simulink model "uas_sim"  (R2020b)
settings: Solver=VariableStepAuto  StartTime=0.0  StopTime=10.0  RelTol=1e-3
undefined symbols (not defined in the file or in its folder): b, c, Earth, InitCond, prop_angle, voltage, WGS84
libraries: aerolibasang x3, aerolibactuator x1, aerolibadyn x1, sharedutil x1, aerolibbdyn x1, sharedtransform x1, shared6dof x1, aerolibconvert2 x1, aerolibtransform2 x1, aerolibgravity2 x1
settings Model: Creator=brian  LastModifiedBy=brian

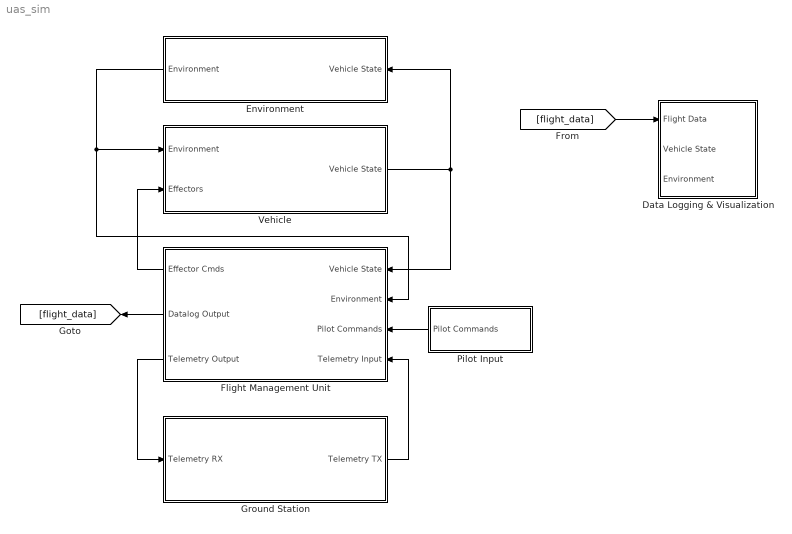
== system uas_sim ==
  Data Logging & Visualization : Subsystem
  Environment : Subsystem
  Flight Management Unit : Subsystem
  Ground Station : Subsystem
  Pilot Input : Subsystem
  Vehicle : Subsystem
  wires:
  Vehicle/1(Vehicle State) -> Flight Management Unit/1(Vehicle State), Environment/1(Vehicle State)
  Pilot Input/1(Pilot Commands) -> Flight Management Unit/3(Pilot Commands)
  Ground Station/1(Telemetry TX) -> Flight Management Unit/4(Telemetry Input)
  Flight Management Unit/3(Telemetry Output) -> Ground Station/1(Telemetry RX)
  Flight Management Unit/1(Effector Cmds) -> Vehicle/2(Effectors)
  [flight_data] -> Data Logging & Visualization/1(Flight Data)
  Flight Management Unit/2(Datalog Output) -> [flight_data]
  Environment/1(Environment) -> Vehicle/1(Environment), Flight Management Unit/2(Environment)

== system uas_sim/Data Logging & Visualization ==
  Flight Data : Inport
  Vehicle State : Inport  Port=2
  Environment : Inport  Port=3

== system uas_sim/Environment ==
  Vehicle State : Inport
  Bus Creator : BusCreator  Inputs=6
  Bus Selector : BusSelector  OutputSignals=Latitude [rad],Longitude [rad],Altitude WGS84 [m]
  Model : ModelReference  ModelNameDialog=env_mdl_aero_blockset.slx  SimulationMode=Normal  ModelReferenceVersion=1.5
  Environment : Outport
  wires:
  Vehicle State/1 -> Bus Selector/1
  Bus Selector/1 -> Model/1  "<Latitude [rad]>"
  Bus Selector/2 -> Model/2  "<Longitude [rad]>"
  Bus Selector/3 -> Model/3  "<Altitude WGS84 [m]>"
  Bus Creator/1 -> Environment/1
  Model/3 -> Bus Creator/3  "Pressure [Pa]"
  Model/2 -> Bus Creator/2  "Speed of Sound [m/s]"
  Model/1 -> Bus Creator/1  "Temperature [K]"
  Model/4 -> Bus Creator/4  "Density [kg/m^3]"
  Model/5 -> Bus Creator/5  "Gravity [m/s/s]"
  Model/6 -> Bus Creator/6  "Magnetic Field [uT]"

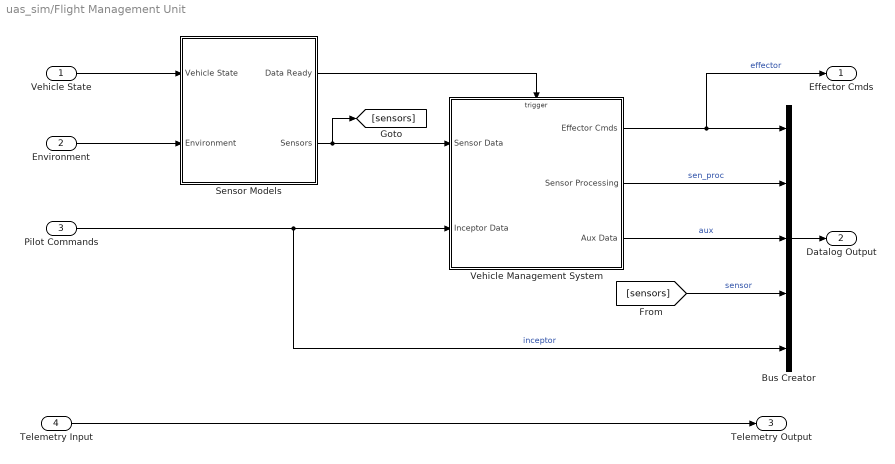
== system uas_sim/Flight Management Unit ==
  Vehicle State : Inport
  Environment : Inport  Port=2
  Pilot Commands : Inport  Port=3  OutDataTypeStr=Bus: InceptorData
  Telemetry Input : Inport  Port=4
  Bus Creator : BusCreator  Inputs=5
  Sensor Models : Subsystem
      settings: PortSchema="{\"entries\":[{\"content\":{\"sides\":[{\"content\":{\"connectorIds\":[]},\"type\":\"ConnectorPlacement.EquallySpacedRectSide\",\"uuid\":\"b20f7590-d69b-48b8-beb1-2fb7d3ab0357\"},{\"content\":{\"connectorIds\":[],\"side\":\"RIGHT\"},\"type\":\"ConnectorPlacement.EquallySpacedRectSide\",\"uuid\":\"07801f8a-7756-483e-a050-3c2fccc33404\"},{\"content\":{\"connectorIds\":[\"In1\",\"In2\"],\"side\":\"TOP\"},\"type\":\"ConnectorPlacement.EquallySpacedRectSide\",\"uuid\":\"ce3c3c94-ed36-4103-b079-69dcaeaf21e9\"},{\"content\":{\"connectorIds\":[\"Out1\",\"Out2\"],\"side\":\"BOTTOM\"},\"type\":\"ConnectorPlacement.EquallySpacedRectSide\",\"uuid\":\"ba78b819-a471-4bc3-b479-e6a973cfe14f\"},{\"content\":{\"connectorIds\":[],\"side\":\"HIDDEN\"},\"type\":\"ConnectorPlacement.EquallySpacedRectSide\",\"uuid\":\"3cf915a5-25a1-4380-9090-9561533312da\"}]},\"type\":\"ConnectorPlacement.EquallySpacedConnector\",\"uuid\":\"7ef4ddaa-ccd2-4778-89ce-8b4685524e82\"}],\"packageUris\":[\"http://schema.mathworks.com/mf0/Connector/R2020b\"],\"version\":\"1.0\"}"
  Vehicle Management System : Subsystem  TreatAsAtomicUnit=on
  Effector Cmds : Outport  OutDataTypeStr=Bus: EffectorCmds
  Datalog Output : Outport  Port=2
  Telemetry Output : Outport  Port=3
  wires:
  Telemetry Input/1 -> Telemetry Output/1
  Pilot Commands/1 -> Bus Creator/5, Vehicle Management System/2(Inceptor Data)  "inceptor"
  Sensor Models/2(Data Ready) -> Vehicle Management System/Trigger
  Bus Creator/1 -> Datalog Output/1
  Vehicle Management System/3(Aux Data) -> Bus Creator/3  "aux"
  Vehicle Management System/1(Effector Cmds) -> Effector Cmds/1, Bus Creator/1  "effector"
  Vehicle Management System/2(Sensor Processing) -> Bus Creator/2  "sen_proc"
  Environment/1 -> Sensor Models/1(Environment)
  Vehicle State/1 -> Sensor Models/2(Vehicle State)
  Sensor Models/1(Sensors) -> [sensors], Vehicle Management System/1(Sensor Data)
  [sensors] -> Bus Creator/4  "sensor"

== system uas_sim/Ground Station ==
  Telemetry RX : Inport
  Telemetry TX : Outport
  wires:
  Telemetry RX/1 -> Telemetry TX/1

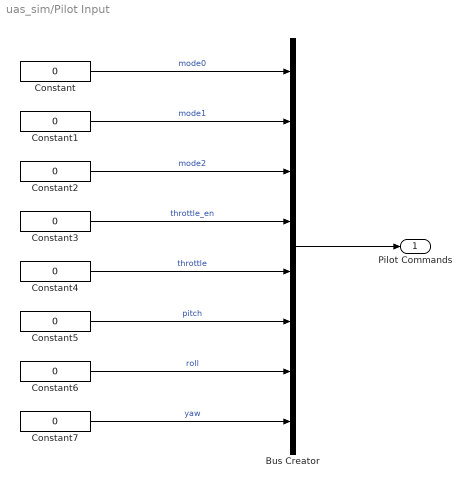
== system uas_sim/Pilot Input ==
  Bus Creator : BusCreator  Inputs=8
  Constant{,1..7} (8 alike) : Constant  Value=0
  Pilot Commands : Outport  OutDataTypeStr=Bus: InceptorData
  wires:
  Bus Creator/1 -> Pilot Commands/1
  Constant/1 -> Bus Creator/1  "mode0"
  Constant1/1 -> Bus Creator/2  "mode1"
  Constant2/1 -> Bus Creator/3  "mode2"
  Constant3/1 -> Bus Creator/4  "throttle_en"
  Constant4/1 -> Bus Creator/5  "throttle"
  Constant5/1 -> Bus Creator/6  "pitch"
  Constant6/1 -> Bus Creator/7  "roll"
  Constant7/1 -> Bus Creator/8  "yaw"

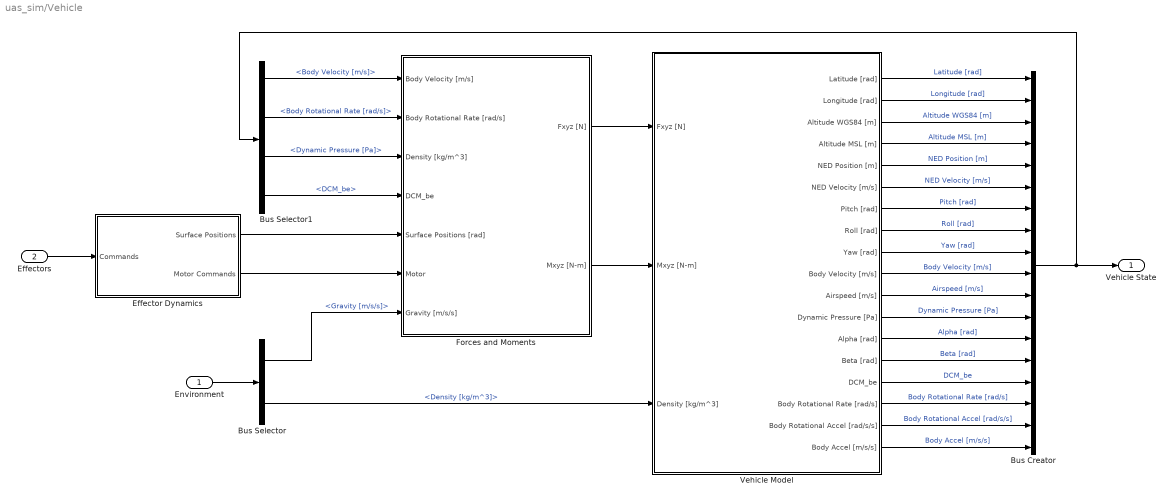
== system uas_sim/Vehicle ==
  Environment : Inport
  Effectors : Inport  Port=2
  Bus Creator : BusCreator  Inputs=18
  Bus Selector : BusSelector  OutputSignals=Gravity [m/s/s],Density [kg/m^3]
  Bus Selector1 : BusSelector  OutputSignals=Body Velocity [m/s],Body Rotational Rate [rad/s],Dynamic Pressure [Pa],DCM_be
  Effector Dynamics : Subsystem
      settings: PortSchema="{\"entries\":[{\"content\":{\"sides\":[{\"content\":{\"connectorIds\":[]},\"type\":\"ConnectorPlacement.EquallySpacedRectSide\",\"uuid\":\"b20f7590-d69b-48b8-beb1-2fb7d3ab0357\"},{\"content\":{\"connectorIds\":[],\"side\":\"RIGHT\"},\"type\":\"ConnectorPlacement.EquallySpacedRectSide\",\"uuid\":\"07801f8a-7756-483e-a050-3c2fccc33404\"},{\"content\":{\"connectorIds\":[\"Out1\",\"Out2\"],\"side\":\"TOP\"},\"type\":\"ConnectorPlacement.EquallySpacedRectSide\",\"uuid\":\"ce3c3c94-ed36-4103-b079-69dcaeaf21e9\"},{\"content\":{\"connectorIds\":[\"In1\"],\"side\":\"BOTTOM\"},\"type\":\"ConnectorPlacement.EquallySpacedRectSide\",\"uuid\":\"ba78b819-a471-4bc3-b479-e6a973cfe14f\"},{\"content\":{\"connectorIds\":[],\"side\":\"HIDDEN\"},\"type\":\"ConnectorPlacement.EquallySpacedRectSide\",\"uuid\":\"3cf915a5-25a1-4380-9090-9561533312da\"}]},\"type\":\"ConnectorPlacement.EquallySpacedConnector\",\"uuid\":\"7ef4ddaa-ccd2-4778-89ce-8b4685524e82\"}],\"packageUris\":[\"http://schema.mathworks.com/mf0/Connector/R2020b\"],\"version\":\"1.0\"}"
  Forces and Moments : Subsystem
  Vehicle Model : Subsystem
  Vehicle State : Outport
  wires:
  Vehicle Model/1(Latitude [rad]) -> Bus Creator/1  "Latitude [rad]"
  Vehicle Model/2(Longitude [rad]) -> Bus Creator/2  "Longitude [rad]"
  Vehicle Model/3(Altitude WGS84 [m]) -> Bus Creator/3  "Altitude WGS84 [m]"
  Vehicle Model/4(Altitude MSL [m]) -> Bus Creator/4  "Altitude MSL [m]"
  Vehicle Model/5(NED Position [m]) -> Bus Creator/5  "NED Position [m]"
  Vehicle Model/6(NED Velocity [m/s]) -> Bus Creator/6  "NED Velocity [m/s]"
  Vehicle Model/7(Pitch [rad]) -> Bus Creator/7  "Pitch [rad]"
  Vehicle Model/8(Roll [rad]) -> Bus Creator/8  "Roll [rad]"
  Vehicle Model/9(Yaw [rad]) -> Bus Creator/9  "Yaw [rad]"
  Vehicle Model/12(Dynamic Pressure [Pa]) -> Bus Creator/12  "Dynamic Pressure [Pa]"
  Vehicle Model/13(Alpha [rad]) -> Bus Creator/13  "Alpha [rad]"
  Vehicle Model/14(Beta [rad]) -> Bus Creator/14  "Beta [rad]"
  Vehicle Model/15(DCM_be) -> Bus Creator/15  "DCM_be"
  Vehicle Model/16(Body Rotational Rate [rad/s]) -> Bus Creator/16  "Body Rotational Rate [rad/s]"
  Vehicle Model/17(Body Rotational Accel [rad/s/s]) -> Bus Creator/17  "Body Rotational Accel [rad/s/s]"
  Vehicle Model/18(Body Accel [m/s/s]) -> Bus Creator/18  "Body Accel [m/s/s]"
  Effectors/1 -> Effector Dynamics/1(Commands)
  Effector Dynamics/1(Surface Positions) -> Forces and Moments/5(Surface Positions [rad])
  Effector Dynamics/2(Motor Commands) -> Forces and Moments/6(Motor)
  Environment/1 -> Bus Selector/1
  Bus Selector/1 -> Forces and Moments/7(Gravity [m/s/s])  "<Gravity [m/s/s]>"
  Bus Selector/2 -> Vehicle Model/3(Density [kg/m^3])  "<Density [kg/m^3]>"
  Bus Creator/1 -> Bus Selector1/1, Vehicle State/1
  Vehicle Model/11(Airspeed [m/s]) -> Bus Creator/11  "Airspeed [m/s]"
  Bus Selector1/4 -> Forces and Moments/4(DCM_be)  "<DCM_be>"
  Vehicle Model/10(Body Velocity [m/s]) -> Bus Creator/10  "Body Velocity [m/s]"
  Bus Selector1/1 -> Forces and Moments/1(Body Velocity [m/s])  "<Body Velocity [m/s]>"
  Bus Selector1/2 -> Forces and Moments/2(Body Rotational Rate [rad/s])  "<Body Rotational Rate [rad/s]>"
  Bus Selector1/3 -> Forces and Moments/3(Density [kg/m^3])  "<Dynamic Pressure [Pa]>"
  Forces and Moments/1(Fxyz [N]) -> Vehicle Model/1(Fxyz [N])
  Forces and Moments/2(Mxyz [N-m]) -> Vehicle Model/2(Mxyz [N-m])

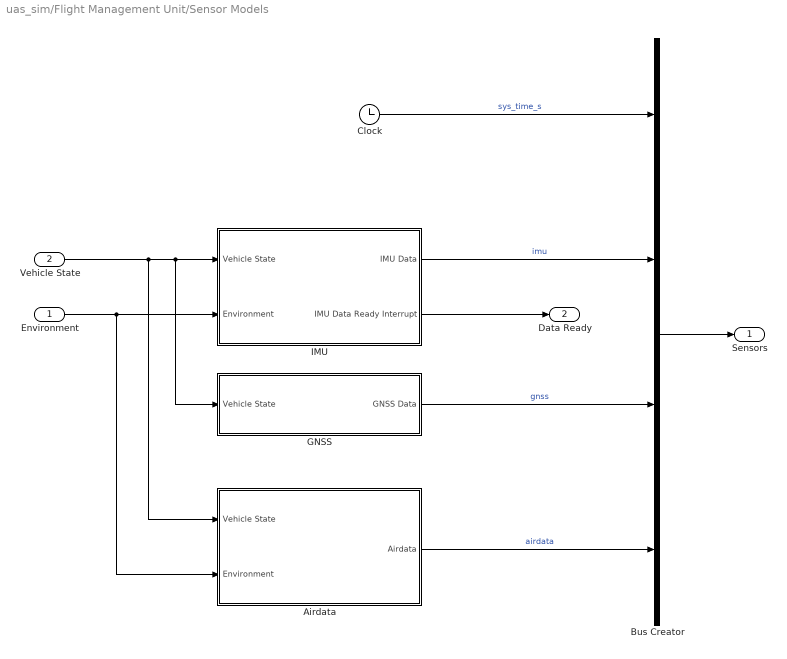
== system uas_sim/Flight Management Unit/Sensor Models ==
  Environment : Inport
  Vehicle State : Inport  Port=2
  Airdata : Subsystem
  Bus Creator : BusCreator  Inputs=4  OutDataTypeStr=Bus: SensorData  NonVirtualBus=on
      settings: InheritFromInputs=off
  Clock : Clock
      settings: Decimation=1e6
  GNSS : Subsystem
  IMU : Subsystem
  Sensors : Outport
  Data Ready : Outport  Port=2
  wires:
  Bus Creator/1 -> Sensors/1
  Clock/1 -> Bus Creator/1  "sys_time_s"
  IMU/1(IMU Data) -> Bus Creator/2  "imu"
  IMU/2(IMU Data Ready Interrupt) -> Data Ready/1
  Vehicle State/1 -> Airdata/1(Vehicle State), GNSS/1(Vehicle State), IMU/1(Vehicle State)
  Environment/1 -> Airdata/2(Environment), IMU/2(Environment)
  GNSS/1(GNSS Data) -> Bus Creator/3  "gnss"
  Airdata/1(Airdata) -> Bus Creator/4  "airdata"

== system uas_sim/Flight Management Unit/Vehicle Management System ==
  Sensor Data : Inport  OutDataTypeStr=Bus: SensorData
  Inceptor Data : Inport  Port=2  OutDataTypeStr=Bus: SenProcData
  Trigger : TriggerPort  VariantControl=Variant
  Model : ModelReference  ModelNameDialog=baseline.slx  SimulationMode=Normal  ModelReferenceVersion=1.11
  Effector Cmds : Outport  OutDataTypeStr=Bus: EffectorCmds
  Sensor Processing : Outport  Port=2  OutDataTypeStr=Bus: SenProcData
  Aux Data : Outport  Port=3  OutDataTypeStr=Bus: AuxData
  wires:
  Model/2 -> Sensor Processing/1
  Model/3 -> Aux Data/1
  Model/1 -> Effector Cmds/1
  Sensor Data/1 -> Model/1
  Inceptor Data/1 -> Model/2

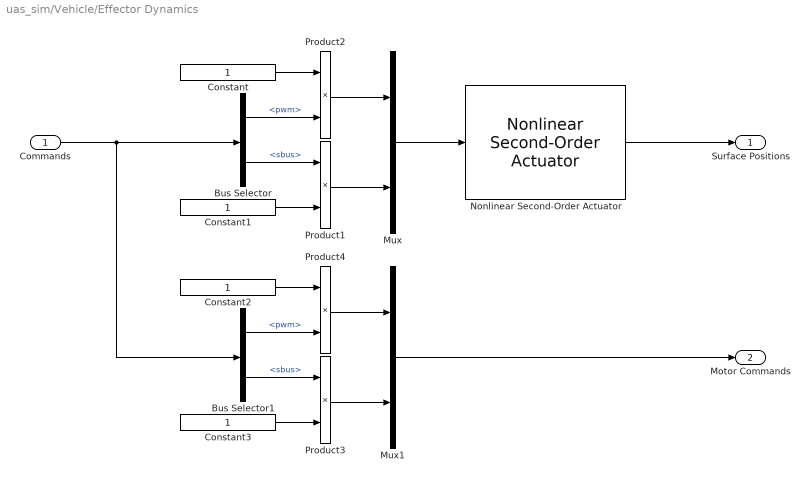
== system uas_sim/Vehicle/Effector Dynamics ==
  Commands : Inport
  Bus Selector : BusSelector  OutputSignals=pwm,sbus
  Bus Selector1 : BusSelector  OutputSignals=pwm,sbus
  Constant{,1..3} (4 alike) : Constant
  Mux : Mux  Inputs=2
  Mux1 : Mux  Inputs=2
  Nonlinear Second-Order Actuator : aerolibactuator/Nonlinear Second-Order Actuator  wn_fin=1  z_fin=0.3  fin_max=20*pi/180  fin_min=-20*pi/180  fin_maxrate=500*pi/180  fin_act_0=0  fin_act_vel=0
      settings: SourceProductBaseCode=AE
  Product{1..4} (4 alike) : Product
  Surface Positions : Outport
  Motor Commands : Outport  Port=2
  wires:
  Commands/1 -> Bus Selector1/1, Bus Selector/1
  Bus Selector/1 -> Product2/2  "<pwm>"
  Bus Selector/2 -> Product1/1  "<sbus>"
  Mux/1 -> Nonlinear Second-Order Actuator/1
  Nonlinear Second-Order Actuator/1 -> Surface Positions/1
  Product2/1 -> Mux/1
  Product1/1 -> Mux/2
  Constant/1 -> Product2/1
  Constant1/1 -> Product1/2
  Constant3/1 -> Product3/2
  Constant2/1 -> Product4/1
  Product3/1 -> Mux1/2
  Product4/1 -> Mux1/1
  Mux1/1 -> Motor Commands/1
  Bus Selector1/2 -> Product3/1  "<sbus>"
  Bus Selector1/1 -> Product4/2  "<pwm>"

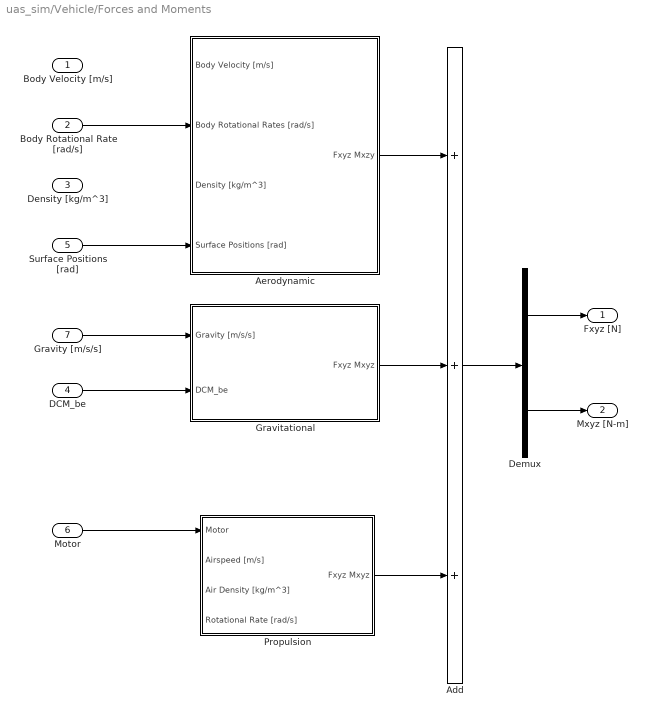
== system uas_sim/Vehicle/Forces and Moments ==
  Body Velocity [m/s] : Inport
  Body Rotational Rate [rad/s] : Inport  Port=2
  Density [kg/m^3] : Inport  Port=3
  DCM_be : Inport  Port=4
  Surface Positions [rad] : Inport  Port=5
  Motor : Inport  Port=6
  Gravity [m/s/s] : Inport  Port=7
  Add : Sum  Inputs=+++
  Aerodynamic : Subsystem
  Demux : Demux  Outputs=2
  Gravitational : Subsystem
  Propulsion : Subsystem
  Fxyz [N] : Outport
  Mxyz [N-m] : Outport  Port=2
  wires:
  Surface Positions [rad]/1 -> Aerodynamic/4(Surface Positions [rad])
  Body Rotational Rate [rad/s]/1 -> Aerodynamic/2(Body Rotational Rates [rad/s])
  Gravitational/1(Fxyz Mxyz) -> Add/2
  Aerodynamic/1(Fxyz Mxzy) -> Add/1
  Propulsion/1(Fxyz Mxyz) -> Add/3
  Gravity [m/s/s]/1 -> Gravitational/1(Gravity [m/s/s])
  DCM_be/1 -> Gravitational/2(DCM_be)
  Motor/1 -> Propulsion/1(Motor)
  Add/1 -> Demux/1
  Demux/2 -> Mxyz [N-m]/1
  Demux/1 -> Fxyz [N]/1

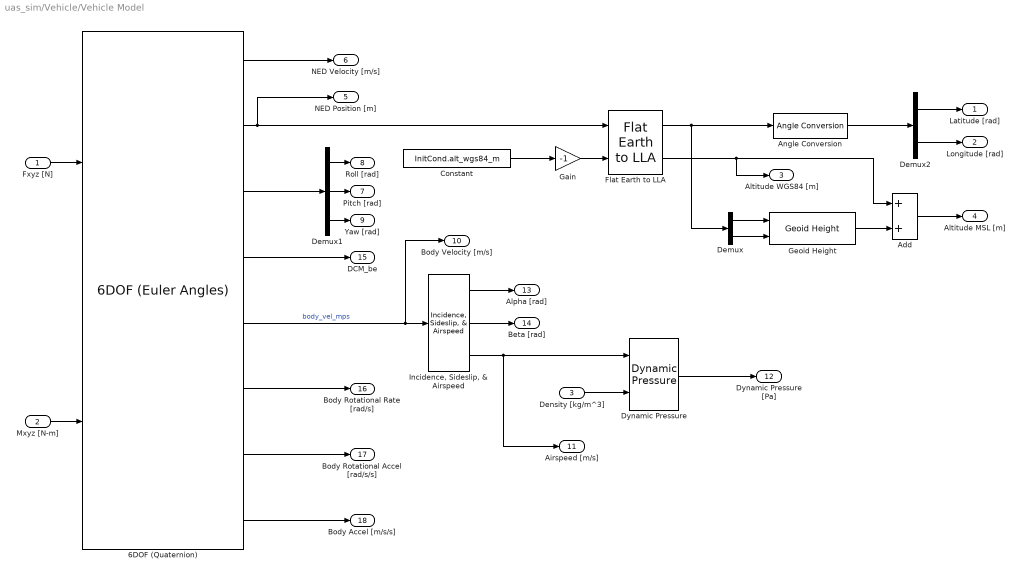
== system uas_sim/Vehicle/Vehicle Model ==
  Fxyz [N] : Inport
  Mxyz [N-m] : Inport  Port=2
  Density [kg/m^3] : Inport  Port=3
  6DOF (Quaternion) : shared6dof/6DOF (Euler Angles)  units=Metric (MKS)  mtype=Fixed  rep=Euler Angles  xme_0=[0 0 0]  Vm_0=[InitCond.vel_u_mps InitCond.vel_v_mps InitCond.vel_w_mps]  eul_0=[InitCond.roll_rad InitCond.pitch_rad InitCond.yaw_rad]  pm_0=[InitCond.p_radps InitCond.q_rads InitCond.r_radps]  mass_0=Aircraft.Mass.mass_kg  mass_e=0.5  mass_f=2.0  inertia=Aircraft.Mass.inertia_kgm2  inertia_e=eye(3)  inertia_f=2*eye(3)  k_quat=1.0  vre_flag=on  abi_flag=off  aMode=0  xme_statename=''  Vm_statename=''  eul_statename=''  quat_statename=''  pm_statename=''  mass_statename=''
      settings: SourceProductBaseCode=AE,PW,MT,UV,VE,VP
  Add : Sum
  Angle Conversion : aerolibconvert2/Angle Conversion  IU=deg  OU=rad
  Constant : Constant  Value=InitCond.alt_wgs84_m
  Demux : Demux  Outputs=2
  Demux1 : Demux  Outputs=3
  Demux2 : Demux  Outputs=2
  Dynamic Pressure : aerolibasang/Dynamic Pressure
  Flat Earth to LLA : aerolibtransform2/Flat Earth to LLA  units=Metric (MKS)  ptype=Earth (WGS84)  F=1/298.257223563  R=6378137  refPosPort=off  LL0=[rad2deg(InitCond.lat_rad) rad2deg(InitCond.lon_rad)]  psi=0
  Gain : Gain  Gain=-1
  Geoid Height : aerolibgravity2/Geoid Height  units=Metric (MKS)  gtype=EGM2008  datafile='geoidegm96grid'  dtype=double  action=Warning
      settings: AttributesFormatString=EGM2008 Geoid Data Unavailable  SourceProductBaseCode=AE
  "Incidence, Sideslip, & Airspeed" : aerolibasang/Incidence, Sideslip, & Airspeed
  Latitude [rad] : Outport
  Longitude [rad] : Outport  Port=2
  Altitude WGS84 [m] : Outport  Port=3
  Altitude MSL [m] : Outport  Port=4
  NED Position [m] : Outport  Port=5
  NED Velocity [m/s] : Outport  Port=6
  Pitch [rad] : Outport  Port=7
  Roll [rad] : Outport  Port=8
  Yaw [rad] : Outport  Port=9
  Body Velocity [m/s] : Outport  Port=10
  Airspeed [m/s] : Outport  Port=11
  Dynamic Pressure [Pa] : Outport  Port=12
  Alpha [rad] : Outport  Port=13
  Beta [rad] : Outport  Port=14
  DCM_be : Outport  Port=15
  Body Rotational Rate [rad/s] : Outport  Port=16
  Body Rotational Accel [rad/s/s] : Outport  Port=17
  Body Accel [m/s/s] : Outport  Port=18
  wires:
  Fxyz [N]/1 -> 6DOF (Quaternion)/1
  Mxyz [N-m]/1 -> 6DOF (Quaternion)/2
  6DOF (Quaternion)/2 -> NED Position [m]/1, Flat Earth to LLA/1
  6DOF (Quaternion)/5 -> Body Velocity [m/s]/1, "Incidence, Sideslip, & Airspeed"/1  "body_vel_mps"
  Flat Earth to LLA/1 -> Demux/1, Angle Conversion/1
  Flat Earth to LLA/2 -> Altitude WGS84 [m]/1, Add/1
  Geoid Height/1 -> Add/2
  Demux/2 -> Geoid Height/2
  Demux/1 -> Geoid Height/1
  "Incidence, Sideslip, & Airspeed"/3 -> Airspeed [m/s]/1, Dynamic Pressure/1
  Density [kg/m^3]/1 -> Dynamic Pressure/2
  Angle Conversion/1 -> Demux2/1
  6DOF (Quaternion)/1 -> NED Velocity [m/s]/1
  6DOF (Quaternion)/4 -> DCM_be/1
  Demux1/1 -> Roll [rad]/1
  6DOF (Quaternion)/3 -> Demux1/1
  Demux1/2 -> Pitch [rad]/1
  Demux1/3 -> Yaw [rad]/1
  Dynamic Pressure/1 -> Dynamic Pressure [Pa]/1
  "Incidence, Sideslip, & Airspeed"/1 -> Alpha [rad]/1
  "Incidence, Sideslip, & Airspeed"/2 -> Beta [rad]/1
  Add/1 -> Altitude MSL [m]/1
  Gain/1 -> Flat Earth to LLA/2
  Constant/1 -> Gain/1
  Demux2/2 -> Longitude [rad]/1
  Demux2/1 -> Latitude [rad]/1
  6DOF (Quaternion)/6 -> Body Rotational Rate [rad/s]/1
  6DOF (Quaternion)/7 -> Body Rotational Accel [rad/s/s]/1
  6DOF (Quaternion)/8 -> Body Accel [m/s/s]/1

== system uas_sim/Flight Management Unit/Sensor Models/Airdata ==
  Vehicle State : Inport
  Environment : Inport  Port=2
  Bus Creator : BusCreator  Inputs=2
  Bus Selector : BusSelector  OutputSignals=Dynamic Pressure [Pa]
  Bus Selector1 : BusSelector  OutputSignals=Pressure [Pa]
  Model : ModelReference  ModelNameDialog=pressure.slx  UsingDefaultArgumentValue=0,0,0,0,0,0  SimulationMode=Normal  ModelReferenceVersion=1.10  scale=Sensors.DiffPres.scale_factor  bias=Sensors.DiffPres.bias_pa  noise=Sensors.DiffPres.noise_pa  p_sath=Sensors.DiffPres.upper_limit_pa  p_satl=Sensors.DiffPres.lower_limit_pa  sample_rate=Sensors.DiffPres.sample_rate_hz  SimulationMode=Normal
  Model1 : ModelReference  ModelNameDialog=pressure.slx  UsingDefaultArgumentValue=0,0,0,0,0,0  SimulationMode=Normal  ModelReferenceVersion=1.10  scale=Sensors.StaticPres.scale_factor  bias=Sensors.StaticPres.bias_pa  noise=Sensors.StaticPres.noise_pa  p_sath=Sensors.StaticPres.upper_limit_pa  p_satl=Sensors.StaticPres.lower_limit_pa  sample_rate=Sensors.StaticPres.sample_rate_hz  SimulationMode=Normal
  Airdata : Outport  OutDataTypeStr=Bus: AirData
  wires:
  Vehicle State/1 -> Bus Selector/1
  Bus Selector/1 -> Model/1  "<Dynamic Pressure [Pa]>"
  Model/1 -> Bus Creator/1  "diff_pres_pa"
  Bus Creator/1 -> Airdata/1
  Model1/1 -> Bus Creator/2  "static_pres_pa"
  Environment/1 -> Bus Selector1/1
  Bus Selector1/1 -> Model1/1  "<Pressure [Pa]>"

== system uas_sim/Flight Management Unit/Sensor Models/GNSS ==
  Vehicle State : Inport
  Bus Creator : BusCreator  Inputs=13  OutDataTypeStr=Bus: GnssData
      settings: InheritFromInputs=off
  Bus Selector : BusSelector  OutputSignals=Latitude [rad],Longitude [rad],Altitude WGS84 [m],NED Velocity [m/s]
  Demux : Demux  Outputs=3
  Model : ModelReference  ModelNameDialog=gnss_receiver.slx  UsingDefaultArgumentValue=0,0,0,0,0  SimulationMode=Normal  ModelReferenceVersion=1.25  fix=Sensors.Gnss.fix  num_sat=Sensors.Gnss.num_satellites  pos_acc_m=Sensors.Gnss.pos_accuracy_m  vel_acc_mps=Sensors.Gnss.vel_accuracy_mps  sample_rate=Sensors.Gnss.sample_rate_hz  SimulationMode=Normal
  GNSS Data : Outport  OutDataTypeStr=Bus: GnssData
  wires:
  Vehicle State/1 -> Bus Selector/1
  Bus Selector/1 -> Model/1  "<Latitude [rad]>"
  Bus Selector/2 -> Model/2  "<Longitude [rad]>"
  Bus Selector/3 -> Model/3  "<Altitude WGS84 [m]>"
  Bus Selector/4 -> Model/4  "<NED Velocity [m/s]>"
  Bus Creator/1 -> GNSS Data/1
  Model/1 -> Bus Creator/1  "fix"
  Model/2 -> Bus Creator/2  "num_sats"
  Model/3 -> Bus Creator/3  "tow_s"
  Model/4 -> Bus Creator/4  "week"
  Model/5 -> Bus Creator/5  "lat_rad"
  Model/6 -> Bus Creator/6  "lon_rad"
  Model/7 -> Bus Creator/7  "alt_wgs84_m"
  Model/11 -> Bus Creator/13  "vel_acc_mps"
  Model/10 -> Bus Creator/12  "vert_acc_m"
  Model/9 -> Bus Creator/11  "horz_acc_m"
  Demux/2 -> Bus Creator/9  "ned_vel_y_mps"
  Demux/1 -> Bus Creator/8  "ned_vel_x_mps"
  Demux/3 -> Bus Creator/10  "ned_vel_z_mps"
  Model/8 -> Demux/1

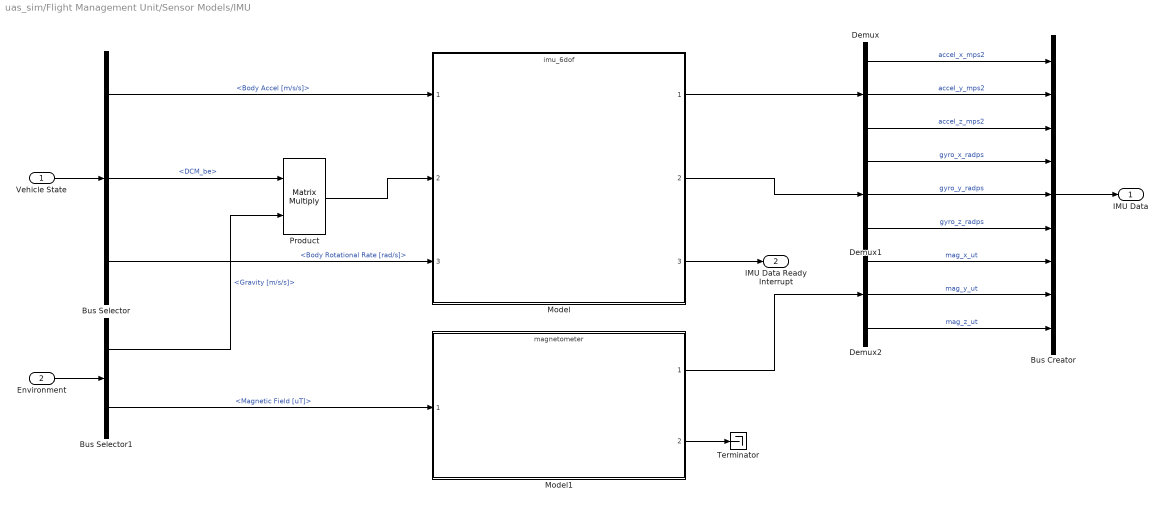
== system uas_sim/Flight Management Unit/Sensor Models/IMU ==
  Vehicle State : Inport
  Environment : Inport  Port=2
  Bus Creator : BusCreator  Inputs=9  OutDataTypeStr=Bus: ImuData
      settings: InheritFromInputs=off
  Bus Selector : BusSelector  OutputSignals=Body Accel [m/s/s],DCM_be,Body Rotational Rate [rad/s]
  Bus Selector1 : BusSelector  OutputSignals=Gravity [m/s/s],Magnetic Field [uT]
  Demux : Demux  Outputs=3
  Demux1 : Demux  Outputs=3
  Demux2 : Demux  Outputs=3
  Model : ModelReference  ModelNameDialog=imu_6dof.slx  UsingDefaultArgumentValue=0,0,0,0,0,0,0,0,0,0,0,0  SimulationMode=Normal  ModelReferenceVersion=1.19  sample_rate=Sensors.Imu.sample_rate_hz  a_sf_cc=Sensors.Imu.Accel.scale_factor  a_bias=Sensors.Imu.Accel.bias_mps2  a_noise=Sensors.Imu.Accel.noise_mps2  a_sath=Sensors.Imu.Accel.upper_limit_mps2  a_satl=Sensors.Imu.Accel.lower_limit_mps2  g_sf_cc=Sensors.Imu.Gyro.scale_factor  g_sen=Sensors.Imu.Gyro.accel_sens_radps  g_bias=Sensors.Imu.Gyro.bias_radps  g_noise=Sensors.Imu.Gyro.noise_radps  g_sath=Sensors.Imu.Gyro.upper_limit_radps  g_satl=Sensors.Imu.Gyro.lower_limit_radps  SimulationMode=Normal
  Model1 : ModelReference  ModelNameDialog=magnetometer.slx  UsingDefaultArgumentValue=0,0,0,0,0,0  SimulationMode=Normal  ModelReferenceVersion=1.24  m_sf_cc=Sensors.Imu.Mag.scale_factor  m_bias=Sensors.Imu.Mag.bias_ut  m_noise=Sensors.Imu.Mag.noise_ut  m_sath=Sensors.Imu.Mag.upper_limit_ut  m_satl=Sensors.Imu.Mag.lower_limit_ut  sample_rate=Sensors.Imu.mag.sample_rate_hz  SimulationMode=Normal
  Product : Product  Multiplication=Matrix(*)
  Terminator : Terminator
  IMU Data : Outport  OutDataTypeStr=Bus: ImuData
  IMU Data Ready Interrupt : Outport  Port=2
  wires:
  Vehicle State/1 -> Bus Selector/1
  Bus Selector/1 -> Model/1  "<Body Accel [m/s/s]>"
  Bus Selector/3 -> Model/3  "<Body Rotational Rate [rad/s]>"
  Environment/1 -> Bus Selector1/1
  Bus Selector/2 -> Product/1  "<DCM_be>"
  Bus Selector1/1 -> Product/2  "<Gravity [m/s/s]>"
  Product/1 -> Model/2
  Bus Selector1/2 -> Model1/1  "<Magnetic Field [uT]>"
  Demux/1 -> Bus Creator/1  "accel_x_mps2"
  Demux/2 -> Bus Creator/2  "accel_y_mps2"
  Demux/3 -> Bus Creator/3  "accel_z_mps2"
  Demux1/1 -> Bus Creator/4  "gyro_x_radps"
  Demux1/2 -> Bus Creator/5  "gyro_y_radps"
  Demux1/3 -> Bus Creator/6  "gyro_z_radps"
  Demux2/3 -> Bus Creator/9  "mag_z_ut"
  Demux2/2 -> Bus Creator/8  "mag_y_ut"
  Demux2/1 -> Bus Creator/7  "mag_x_ut"
  Model/1 -> Demux/1
  Model/2 -> Demux1/1
  Model1/1 -> Demux2/1
  Model/3 -> IMU Data Ready Interrupt/1
  Model1/2 -> Terminator/1
  Bus Creator/1 -> IMU Data/1

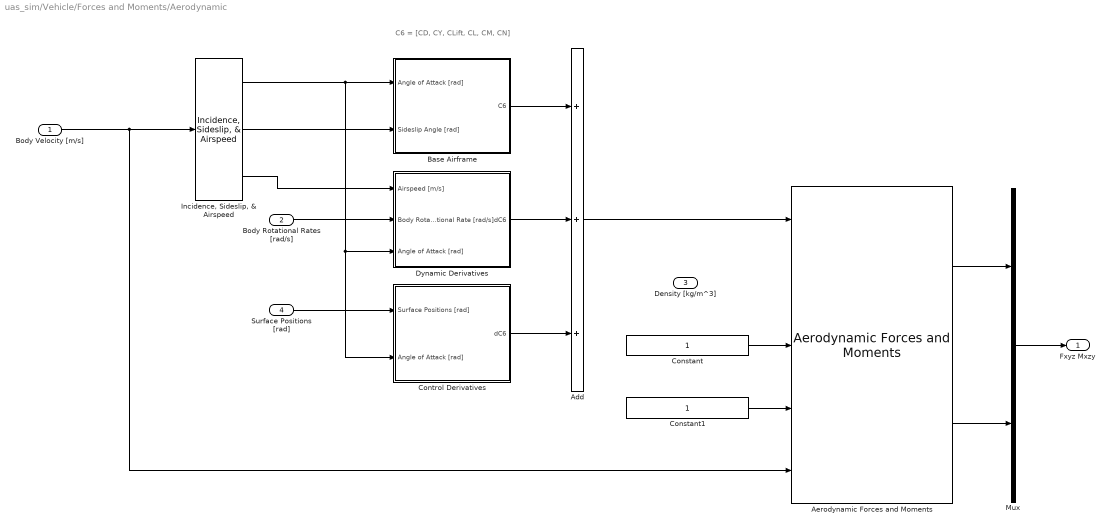
== system uas_sim/Vehicle/Forces and Moments/Aerodynamic ==
  note: C6 = [CD, CY, CLift, CL, CM, CN]
  Body Velocity [m/s] : Inport
  Body Rotational Rates [rad/s] : Inport  Port=2
  Density [kg/m^3] : Inport  Port=3
  Surface Positions [rad] : Inport  Port=4
  Add : Sum  Inputs=+++
  "Aerodynamic Forces and Moments " : aerolibadyn/Aerodynamic Forces and Moments   inputAxes=Wind  outputForceAxes=Body  outputMomentAxes=Body  S=1  b=1  cbar=1
  Base Airframe : Subsystem
  Constant : Constant
  Constant1 : Constant
  Control Derivatives : Subsystem
  Dynamic Derivatives : Subsystem
  "Incidence, Sideslip, & Airspeed" : aerolibasang/Incidence, Sideslip, & Airspeed
  Mux : Mux  Inputs=2
  Fxyz Mxzy : Outport
  wires:
  Base Airframe/1(C6) -> Add/1
  Dynamic Derivatives/1(dC6) -> Add/2
  "Incidence, Sideslip, & Airspeed"/2 -> Base Airframe/2(Sideslip Angle [rad])
  "Incidence, Sideslip, & Airspeed"/1 -> Base Airframe/1(Angle of Attack [rad]), Control Derivatives/2(Angle of Attack [rad]), Dynamic Derivatives/3(Angle of Attack [rad])
  Body Rotational Rates [rad/s]/1 -> Dynamic Derivatives/2(Body Rotational Rate [rad/s])
  "Incidence, Sideslip, & Airspeed"/3 -> Dynamic Derivatives/1(Airspeed [m/s])
  Surface Positions [rad]/1 -> Control Derivatives/1(Surface Positions [rad])
  Control Derivatives/1(dC6) -> Add/3
  Add/1 -> "Aerodynamic Forces and Moments "/1
  Constant/1 -> "Aerodynamic Forces and Moments "/3
  Constant1/1 -> "Aerodynamic Forces and Moments "/4
  Body Velocity [m/s]/1 -> "Aerodynamic Forces and Moments "/5, "Incidence, Sideslip, & Airspeed"/1
  "Aerodynamic Forces and Moments "/1 -> Mux/1
  "Aerodynamic Forces and Moments "/2 -> Mux/2
  Mux/1 -> Fxyz Mxzy/1

== system uas_sim/Vehicle/Forces and Moments/Gravitational ==
  Gravity [m/s/s] : Inport
  DCM_be : Inport  Port=2
  Gravity Moment : Constant  Value=[0 0 0]
  Mux : Mux  Inputs=2
  Product : Product
  Product1 : Product
  UAV Mass : Constant
  Fxyz Mxyz : Outport
  wires:
  Gravity [m/s/s]/1 -> Product/1
  UAV Mass/1 -> Product/2
  Product/1 -> Product1/2  "Gravity Force NED [N]"
  DCM_be/1 -> Product1/1
  Product1/1 -> Mux/1  "Gravity Force Body [N]"
  Gravity Moment/1 -> Mux/2
  Mux/1 -> Fxyz Mxyz/1

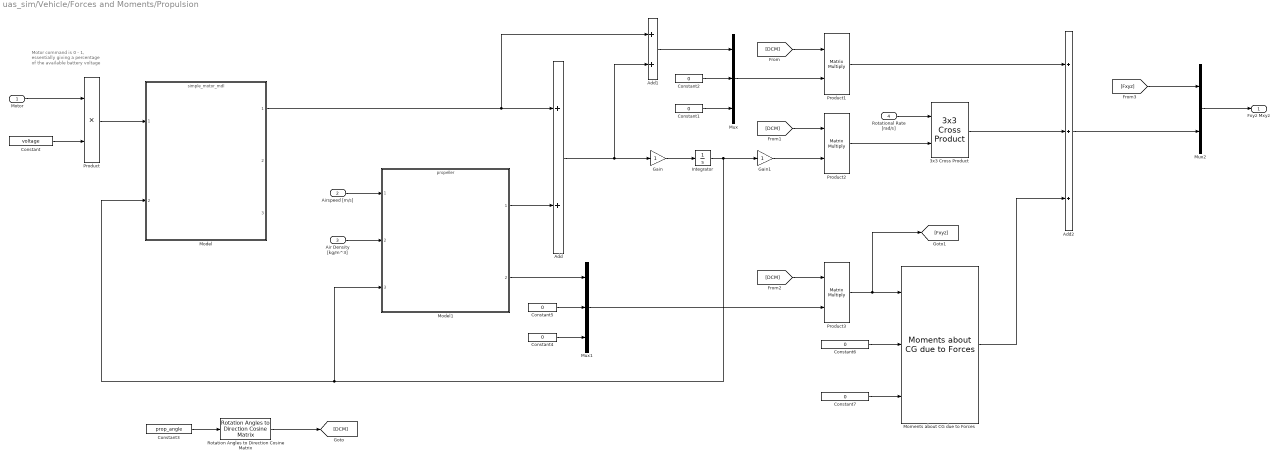
== system uas_sim/Vehicle/Forces and Moments/Propulsion ==
  note: Motor command is 0 - 1,
      | essentially giving a percentage
      | of the available battery voltage
  Motor : Inport
  Airspeed [m/s] : Inport  Port=2
  Air Density [kg/m^3] : Inport  Port=3
  Rotational Rate [rad/s] : Inport  Port=4
  3x3 Cross Product : sharedutil/3x3 Cross Product  aMode=aMode
      settings: SourceProductBaseCode=AE,PW,MT,UV,VE,VP
  Add : Sum
  Add1 : Sum
  Add2 : Sum  Inputs=+++
  Constant : Constant  Value=voltage
  Constant{1..2,4..7} (6 alike) : Constant  Value=0
  Constant3 : Constant  Value=prop_angle
  Gain : Gain
  Gain1 : Gain
  Integrator : Integrator
  Model : ModelReference  ModelNameDialog=simple_motor_mdl.slx  UsingDefaultArgumentValue=0,0,0  SimulationMode=Normal  ModelReferenceVersion=1.4  Kv=670  R=.04  io=3.9  SimulationMode=Normal
  Model1 : ModelReference  ModelNameDialog=propeller.slx  UsingDefaultArgumentValue=0,0,0  SimulationMode=Normal  ModelReferenceVersion=1.9  D=11  Ct=[1 0]  Cp=[1 0]  SimulationMode=Normal
  Moments about CG due to Forces : aerolibbdyn/Moments about CG  due to Forces
      settings: SourceProductBaseCode=AE
  Mux : Mux  Inputs=3
  Mux1 : Mux  Inputs=3
  Mux2 : Mux  Inputs=2
  Product : Product
  Product1 : Product  Multiplication=Matrix(*)
  Product2 : Product  Multiplication=Matrix(*)
  Product3 : Product  Multiplication=Matrix(*)
  Rotation Angles to Direction Cosine Matrix : sharedtransform/Rotation Angles to Direction Cosine Matrix  rotationOrder=ZYX  aMode=aMode
      settings: SourceProductBaseCode=AE,PW,MT,UV,VE,VP
  Fxyz Mxyz : Outport
  wires:
  Product/1 -> Model/1
  Motor/1 -> Product/1
  Constant/1 -> Product/2
  Model1/1 -> Add/2
  Model/1 -> Add1/1, Add/1
  Add/1 -> Add1/2, Gain/1
  Gain/1 -> Integrator/1
  Integrator/1 -> Gain1/1, Model/2, Model1/3
  Constant1/1 -> Mux/3
  Constant2/1 -> Mux/2
  Add1/1 -> Mux/1
  Mux/1 -> Product1/2
  Constant3/1 -> Rotation Angles to Direction Cosine Matrix/1
  Rotation Angles to Direction Cosine Matrix/1 -> [DCM]
  [DCM] -> Product1/1
  [DCM] -> Product2/1
  Gain1/1 -> Product2/2
  Product2/1 -> 3x3 Cross Product/2
  Air Density [kg/m^3]/1 -> Model1/2
  Airspeed [m/s]/1 -> Model1/1
  Rotational Rate [rad/s]/1 -> 3x3 Cross Product/1
  Model1/2 -> Mux1/1
  Constant5/1 -> Mux1/2
  Constant4/1 -> Mux1/3
  [DCM] -> Product3/1
  Mux1/1 -> Product3/2
  Product3/1 -> [Fxyz], Moments about CG due to Forces/1
  3x3 Cross Product/1 -> Add2/2
  Product1/1 -> Add2/1
  Moments about CG due to Forces/1 -> Add2/3
  Add2/1 -> Mux2/2
  Mux2/1 -> Fxyz Mxyz/1
  [Fxyz] -> Mux2/1
  Constant6/1 -> Moments about CG due to Forces/2
  Constant7/1 -> Moments about CG due to Forces/3

== system uas_sim/Vehicle/Forces and Moments/Aerodynamic/Base Airframe ==
  Angle of Attack [rad] : Inport
  Sideslip Angle [rad] : Inport  Port=2
  Constant : Constant  Value=[0:5]
  Interpolation Using Prelookup : Interpolation_n-D  NumberOfTableDimensions=3  NumSelectionDims=1  InternalRulePriority=Speed
      settings: InputPortMap=u0,u1,u2,u3,u4
  Prelookup : PreLookup  BreakpointsData=[10:10:110]  ExtrapMethod=Linear
  Prelookup1 : PreLookup  BreakpointsData=[10:10:110]  ExtrapMethod=Linear
  C6 : Outport
  wires:
  Angle of Attack [rad]/1 -> Prelookup/1
  Prelookup/1 -> Interpolation Using Prelookup/1
  Prelookup/2 -> Interpolation Using Prelookup/2
  Prelookup1/1 -> Interpolation Using Prelookup/3
  Prelookup1/2 -> Interpolation Using Prelookup/4
  Sideslip Angle [rad]/1 -> Prelookup1/1
  Constant/1 -> Interpolation Using Prelookup/5
  Interpolation Using Prelookup/1 -> C6/1

== system uas_sim/Vehicle/Forces and Moments/Aerodynamic/Control Derivatives ==
  note: Look up control effectiveness
  Surface Positions [rad] : Inport
  Angle of Attack [rad] : Inport  Port=2
  Constant : Constant  Value=[0:24]
  Constant1 : Constant  Value=[0:5]
  Interpolation Using Prelookup : Interpolation_n-D  NumberOfTableDimensions=3  NumSelectionDims=2  InternalRulePriority=Speed
  Prelookup1 : PreLookup  BreakpointsData=[10:10:110]  ExtrapMethod=Linear
  Product : Product  Multiplication=Matrix(*)
  dC6 : Outport
  wires:
  Angle of Attack [rad]/1 -> Prelookup1/1
  Prelookup1/2 -> Interpolation Using Prelookup/2
  Prelookup1/1 -> Interpolation Using Prelookup/1
  Surface Positions [rad]/1 -> Product/2
  Interpolation Using Prelookup/1 -> Product/1
  Product/1 -> dC6/1
  Constant1/1 -> Interpolation Using Prelookup/4
  Constant/1 -> Interpolation Using Prelookup/3

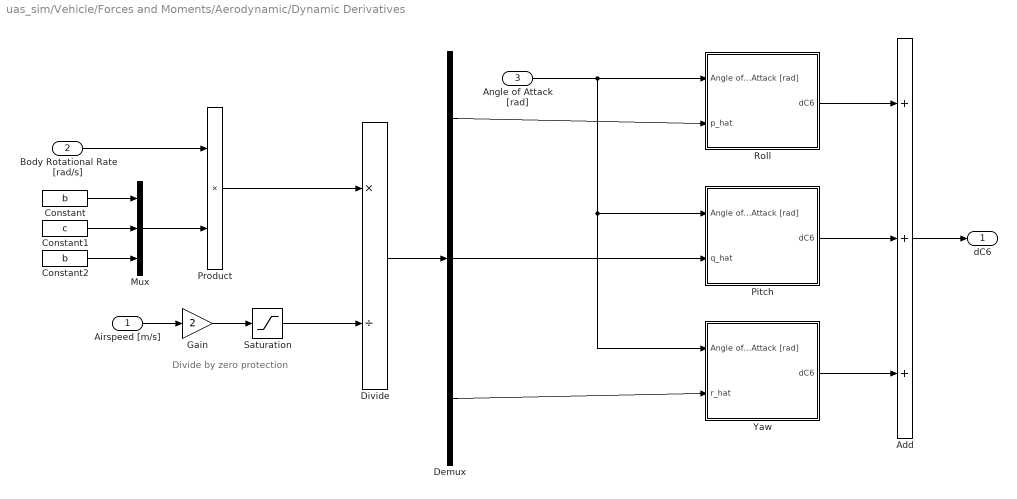
== system uas_sim/Vehicle/Forces and Moments/Aerodynamic/Dynamic Derivatives ==
  note: Divide by zero protection
  Airspeed [m/s] : Inport
  Body Rotational Rate [rad/s] : Inport  Port=2
  Angle of Attack [rad] : Inport  Port=3
  Add : Sum  Inputs=+++
  Constant : Constant  Value=b
  Constant1 : Constant  Value=c
  Constant2 : Constant  Value=b
  Demux : Demux  Outputs=3
  Divide : Product  Inputs=*/
  Gain : Gain  Gain=2
  Mux : Mux  Inputs=3
  Pitch : Subsystem
  Product : Product
  Roll : Subsystem
  Saturation : Saturate  UpperLimit=inf  LowerLimit=1e-3
  Yaw : Subsystem
  dC6 : Outport
  wires:
  Constant/1 -> Mux/1
  Constant1/1 -> Mux/2
  Constant2/1 -> Mux/3
  Body Rotational Rate [rad/s]/1 -> Product/1
  Mux/1 -> Product/2
  Airspeed [m/s]/1 -> Gain/1
  Gain/1 -> Saturation/1
  Product/1 -> Divide/1
  Saturation/1 -> Divide/2
  Divide/1 -> Demux/1
  Demux/1 -> Roll/2(p_hat)
  Demux/2 -> Pitch/2(q_hat)
  Demux/3 -> Yaw/2(r_hat)
  Angle of Attack [rad]/1 -> Yaw/1(Angle of Attack [rad]), Pitch/1(Angle of Attack [rad]), Roll/1(Angle of Attack [rad])
  Roll/1(dC6) -> Add/1
  Pitch/1(dC6) -> Add/2
  Yaw/1(dC6) -> Add/3
  Add/1 -> dC6/1

== system uas_sim/Vehicle/Forces and Moments/Aerodynamic/Dynamic Derivatives/Pitch ==
  Angle of Attack [rad] : Inport
  q_hat : Inport  Port=2
  Constant : Constant  Value=[0:5]
  Interpolation Using Prelookup : Interpolation_n-D  NumberOfTableDimensions=3  NumSelectionDims=1  InternalRulePriority=Speed
      settings: InputPortMap=u0,u1,u2,u3,u4
  Prelookup : PreLookup  BreakpointsData=[10:10:110]  ExtrapMethod=Linear
  Prelookup1 : PreLookup  BreakpointsData=[10:10:110]  ExtrapMethod=Linear
  dC6 : Outport
  wires:
  Prelookup1/1 -> Interpolation Using Prelookup/3
  Prelookup/1 -> Interpolation Using Prelookup/1
  Prelookup/2 -> Interpolation Using Prelookup/2
  Constant/1 -> Interpolation Using Prelookup/5
  Prelookup1/2 -> Interpolation Using Prelookup/4
  Interpolation Using Prelookup/1 -> dC6/1
  Angle of Attack [rad]/1 -> Prelookup1/1
  q_hat/1 -> Prelookup/1

== system uas_sim/Vehicle/Forces and Moments/Aerodynamic/Dynamic Derivatives/Roll ==
  Angle of Attack [rad] : Inport
  p_hat : Inport  Port=2
  Constant : Constant  Value=[0:5]
  Interpolation Using Prelookup : Interpolation_n-D  NumberOfTableDimensions=3  NumSelectionDims=1  InternalRulePriority=Speed
      settings: InputPortMap=u0,u1,u2,u3,u4
  Prelookup : PreLookup  BreakpointsData=[10:10:110]  ExtrapMethod=Linear
  Prelookup1 : PreLookup  BreakpointsData=[10:10:110]  ExtrapMethod=Linear
  dC6 : Outport
  wires:
  Constant/1 -> Interpolation Using Prelookup/5
  Prelookup/1 -> Interpolation Using Prelookup/1
  Prelookup1/1 -> Interpolation Using Prelookup/3
  Prelookup/2 -> Interpolation Using Prelookup/2
  Interpolation Using Prelookup/1 -> dC6/1
  Prelookup1/2 -> Interpolation Using Prelookup/4
  Angle of Attack [rad]/1 -> Prelookup1/1
  p_hat/1 -> Prelookup/1

== system uas_sim/Vehicle/Forces and Moments/Aerodynamic/Dynamic Derivatives/Yaw ==
  Angle of Attack [rad] : Inport
  r_hat : Inport  Port=2
  Constant : Constant  Value=[0:5]
  Interpolation Using Prelookup : Interpolation_n-D  NumberOfTableDimensions=3  NumSelectionDims=1  InternalRulePriority=Speed
      settings: InputPortMap=u0,u1,u2,u3,u4
  Prelookup : PreLookup  BreakpointsData=[10:10:110]  ExtrapMethod=Linear
  Prelookup1 : PreLookup  BreakpointsData=[10:10:110]  ExtrapMethod=Linear
  dC6 : Outport
  wires:
  Prelookup1/1 -> Interpolation Using Prelookup/3
  Prelookup/1 -> Interpolation Using Prelookup/1
  Prelookup/2 -> Interpolation Using Prelookup/2
  Constant/1 -> Interpolation Using Prelookup/5
  Prelookup1/2 -> Interpolation Using Prelookup/4
  Interpolation Using Prelookup/1 -> dC6/1
  Angle of Attack [rad]/1 -> Prelookup1/1
  r_hat/1 -> Prelookup/1
